simulink model "ITRI_Block_fixedQ_Ccode"  (R2017b)
settings: Solver=VariableStepAuto  StartTime=0.0  StopTime=Test_time  RelTol=1e-3
values from neighbouring files (symbols this model uses):
  Lq = L    [mainB_optimization_both.m]    (also in mainC_X_fixedQ_Ccode.m = length(Qnum); mainC_Z_fixedQ_Ccode.m = length(Qnum))
  plant = plantZ_ITRI.v2p    [mainA_itri_pdff.m]    (also in mainB_optimization_both.m = LinearFractionalTransformation(plant); mainC_X_fixedQ_Ccode.m = LinearFractionalTransformation(plant); mainC_Z_fixedQ_Ccode.m = LinearFractionalTransformation(plant))
  Qnum = q    [mainB_optimization_both.m]    (also in mainC_X_fixedQ_Ccode.m = [797.514331990504,-485.232610846030,262.856414138412,24.3359; mainC_Z_fixedQ_Ccode.m = [884.956187600194,-237.650887872230,25.2002633846358,225.998)
  Ts = 0.001    [ID_Model_ITRI.m]
libraries: cstblocks x1
settings Model: Creator=LAB_JHU  LastModifiedBy=LAB_JHU

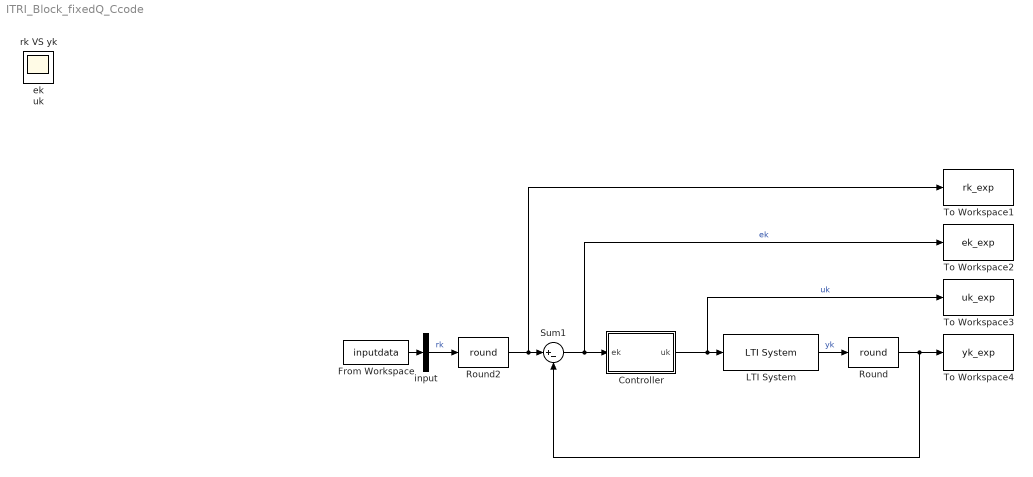
== system ITRI_Block_fixedQ_Ccode ==
  Controller : Subsystem
  From Workspace : FromWorkspace  VariableName=inputdata  SampleTime=Ts
  LTI System : cstblocks/LTI System  sys=plant.v2p  IC=[]
  Round : Rounding  Operator=round
  Round2 : Rounding  Operator=round
  Sum1 : Sum  Inputs=|+-
  To Workspace1 : ToWorkspace  VariableName=rk_exp  SampleTime=-1
  To Workspace2 : ToWorkspace  VariableName=ek_exp  SampleTime=-1
  To Workspace3 : ToWorkspace  VariableName=uk_exp  SampleTime=-1
  To Workspace4 : ToWorkspace  VariableName=yk_exp  SampleTime=-1
  input : Demux  Outputs=1
  ek : Scope
  rk VS yk : Scope
  uk : Scope
  wires:
  Sum1/1 -> To Workspace2/1, Controller/1(ek)  "ek"
  LTI System/1 -> Round/1  "yk"
  Controller/1(uk) -> To Workspace3/1, LTI System/1  "uk"
  input/1 -> Round2/1  "rk"
  From Workspace/1 -> input/1
  Round/1 -> To Workspace4/1, Sum1/2
  Round2/1 -> Sum1/1, To Workspace1/1

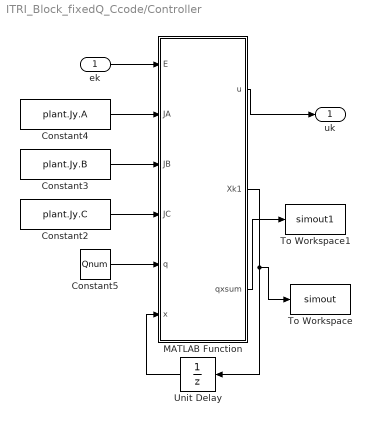
== system ITRI_Block_fixedQ_Ccode/Controller ==
  ek : Inport
  Constant2 : Constant  Value=plant.Jy.C
  Constant3 : Constant  Value=plant.Jy.B
  Constant4 : Constant  Value=plant.Jy.A
  Constant5 : Constant  Value=Qnum
  MATLAB Function : MATLAB Function  TreatAsAtomicUnit=on
  To Workspace : ToWorkspace  VariableName=simout  SampleTime=-1
  To Workspace1 : ToWorkspace  VariableName=simout1  SampleTime=-1
  Unit Delay : UnitDelay  InitialCondition=zeros(Lq+4,1)  SampleTime=-1
  uk : Outport
  wires:
  Constant5/1 -> MATLAB Function/5(q)
  Unit Delay/1 -> MATLAB Function/6(x)
  MATLAB Function/2(Xk1) -> To Workspace/1, Unit Delay/1
  MATLAB Function/1(u) -> uk/1
  ek/1 -> MATLAB Function/1(E)
  Constant4/1 -> MATLAB Function/2(JA)
  Constant3/1 -> MATLAB Function/3(JB)
  Constant2/1 -> MATLAB Function/4(JC)
  MATLAB Function/3(qxsum) -> To Workspace1/1

== matlab function ITRI_Block_fixedQ_Ccode/Controller/MATLAB Function ==
  data: E input; JA input; JB input; JC input; q input; u output; x input; Xk1 output; qxsum output
function [u,Xk1,qxsum] = C_expanded(E,JA,JB,JC,q,x)

q0 = q(1);
qxsum = q(2:length(q)).'*x(6:length(x));

% % general
X0 = (JA(1,:)+JB(1,2)*q0*JC(2,:))*x(1:5) + E*(JB(1,1)+JB(1,2)*q0) + JB(1,2)*qxsum;

X1 = (JA(2,:)+JB(2,2)*q0*JC(2,:))*x(1:5) + E*(JB(2,1)+JB(2,2)*q0) + JB(2,2)*qxsum;

X2 = (JA(3,:)+JB(3,2)*q0*JC(2,:))*x(1:5) + E*(JB(3,1)+JB(3,2)*q0) + JB(3,2)*qxsum;

X3 = (JA(4,:)+JB(4,2)*q0*JC(2,:))*x(1:5) + E*(JB(4,1)+JB(4,2)*q0) + JB(4,2)*qxsum;   

X4 = (JA(5,:)+JB(5,2)*q0*JC(2,:))*x(1:5) + E*(JB(5,1)+JB(5,2)*q0) + JB(5,2)*qxsum;

Z0 = E + JC(2,:)*x(1:5);

Z = x(6:length(x)-1);

Xk1 = [X0; X1; X2; X3; X4; Z0; reshape(Z,[length(Z),1])];

u = (JC(1,:)+q0*JC(2,:))*x(1:5) + E*q0 + qxsum;

end
